simulink model "Motor_ctrl_INST"  (R2024a)
settings: Solver=ode15s  StartTime=0.0  StopTime=1  FixedStep=Ts/10  MaxStep=Tstep  RelTol=1e-3  AbsTol=1e-3  EnableMultiTasking=on
InitFcn:
  | if ~exist('flagwp')
  |     tic
  |     init_sim
  | end
  | mex Motor_ctrl.c User_functions\Src\*.c
StopFcn:
  | if ~exist('flagwp')
  |   elapsed_time=toc
  | end
values from neighbouring files (symbols this model uses):
  accel = 10000    [init_sim.m]
  Bm = 0    [init_sim.m]
  Clarke_inv = [1 0;-0.5 sqrt(3)/2;-0.5 -sqrt(3)/2]    [init_sim.m]
  Ctrl_strategy = 1    [init_sim.m]
  Ctrl_type = 3    [init_sim.m]
  dem = 1    [init_sim.m]
  dT = motorModel.SyreDrive.Converter.dT * 1e-6    [init_sim.m]
  expC = motorModel.IronPMLossMap_dq.expC    [init_sim.m]
  expH = motorModel.IronPMLossMap_dq.expH    [init_sim.m]
  expPM = motorModel.IronPMLossMap_dq.expPM    [init_sim.m]
  fD_pu_norm = motorModel.FluxMapInv_dq.fD_pu_norm    [init_sim.m]
  fD_vct_max = motorModel.FluxMapInv_dq.fD_vct_max    [init_sim.m]
  fD_vct_ref = motorModel.FluxMapInv_dq.fD_vct_ref    [init_sim.m]
  Fm = interp2(Idd,Iqq,Fdd,0,0)    [init_sim.m]
  fQ_pu_norm = motorModel.FluxMapInv_dq.fQ_pu_norm    [init_sim.m]
  fQ_vct_max = motorModel.FluxMapInv_dq.fQ_vct_max    [init_sim.m]
  fQ_vct_ref = motorModel.FluxMapInv_dq.fQ_vct_ref    [init_sim.m]
  HS_ctrl = 1    [init_sim.m]
  Id_dqt = interpn(motorModel.FluxMapInv_dqt.dataF.Fd,motorModel.FluxMapInv_dqt.dataF.Fq,motorModel.FluxMapInv_dqt.dataF.th,motorModel.FluxMapInv_dqt.dataF.Id,Fd_dqt,Fq_dqt,th_dqt,'cubic')    [init_sim.m]
  Id_fe = motorModel.IronPMLossMap_dq.Id    [init_sim.m]
  iD_pu_norm = motorModel.FluxMapInv_dq.iD_pu_norm    [init_sim.m]
  idRef = interp1(abs(MTPA.id+1i*MTPA.iq),MTPA.id,i0)    [init_sim.m]
  InitIntg_d = Fm*cos(th0)    [init_sim.m]
  InitIntg_q = Fm*sin(th0)    [init_sim.m]
  inj_waveform = 1    [init_sim.m]
  Iq_dqt = interpn(motorModel.FluxMapInv_dqt.dataF.Fd,motorModel.FluxMapInv_dqt.dataF.Fq,motorModel.FluxMapInv_dqt.dataF.th,motorModel.FluxMapInv_dqt.dataF.Iq,Fd_dqt,Fq_dqt,th_dqt,'cubic')    [init_sim.m]
  Iq_fe = motorModel.IronPMLossMap_dq.Iq    [init_sim.m]
  iQ_pu_norm = motorModel.FluxMapInv_dq.iQ_pu_norm    [init_sim.m]
  iqRef = interp1(abs(MTPA.id+1i*MTPA.iq),MTPA.iq,i0)    [init_sim.m]
  IronLoss = 1    [init_sim.m]
  J = motorModel.data.J    [init_sim.m]
  motorModelType = motorModel.SyreDrive.modelSetup.motorModelType    [init_sim.m]
  n0 = motorModel.IronPMLossMap_dq.n0    [init_sim.m]
  nRef = 1000    [init_sim.m]
  p = motorModel.data.p    [init_sim.m]
  Pfe_c = motorModel.IronPMLossMap_dq.Pfes_c + motorModel.IronPMLossMap_dq.Pfer_c    [init_sim.m]
  Pfe_h = motorModel.IronPMLossMap_dq.Pfes_h + motorModel.IronPMLossMap_dq.Pfer_h    [init_sim.m]
  Ppm = motorModel.IronPMLossMap_dq.Ppm    [init_sim.m]
  Quad_Maps = 2    [init_sim.m]
  Rs = motorModel.data.Rs    [init_sim.m]
  SS_on = 1    [init_sim.m]
  T_dqt = interpn(motorModel.FluxMapInv_dqt.dataF.Fd,motorModel.FluxMapInv_dqt.dataF.Fq,motorModel.FluxMapInv_dqt.dataF.th,motorModel.FluxMapInv_dqt.dataF.T,Fd_dqt,Fq_dqt,th_dqt,'cubic')    [init_sim.m]
  Tf = 0    [init_sim.m]
  th0 = 0    [init_sim.m]
  th_max = max(motorModel.FluxMapInv_dqt.dataF.th,[],'all')    [init_sim.m]
  th_min = min(motorModel.FluxMapInv_dqt.dataF.th,[],'all')    [init_sim.m]
  Ts = 1/motorModel.SyreDrive.Converter.fPWM    [init_sim.m]
  Tv = 0    [init_sim.m]
  VDC = motorModel.data.Vdc    [init_sim.m]
undefined symbols (not defined in the file or in its folder): ACloss, eMotor, interpn, magnitude, sigbuilder_block, T0
libraries: nesl_utility x52, fl_lib x50, ee_lib x14, simulink x7
(part 4 of 4)

== system Motor_ctrl_INST/Motor model/CCG model/Motor Model/Inverse Flux Maps/3D LUTs/Variant Subsystem/PM-SyR ==
  Fdq : Inport
  theta_elt : Inport  Port=2
  Abs3 : Abs  SaturateOnIntegerOverflow=off
  Demux1 : Demux  Outputs=2
  Interpolation Using Prelookup : Interpolation_n-D  NumberOfTableDimensions=3  Table=T_dqt  LookupTableObject=T_th  RequireIndexFractionAsBus=on  InternalRulePriority=Speed
      settings: InputPortMap=u0,u1,u2
  Interpolation Using Prelookup3 : Interpolation_n-D  NumberOfTableDimensions=3  Table=Id_dqt  RequireIndexFractionAsBus=on  InternalRulePriority=Speed
      settings: InputPortMap=u0,u1,u2
  Interpolation Using Prelookup4 : Interpolation_n-D  NumberOfTableDimensions=3  Table=Iq_dqt  RequireIndexFractionAsBus=on  InternalRulePriority=Speed
      settings: InputPortMap=u0,u1,u2
  MATLAB Function2 : MATLAB Function  TreatAsAtomicUnit=on
  Mux1 : Mux  Inputs=2
  Prelookup1 : PreLookup  BreakpointsData=Fd_v  OutputSelection=Index and fraction as bus  ExtrapMethod=Linear
  Prelookup2 : PreLookup  BreakpointsData=Fq_v  OutputSelection=Index and fraction as bus  ExtrapMethod=Linear
  Prelookup6 : PreLookup  BreakpointsData=th_v  OutputSelection=Index and fraction as bus  ExtrapMethod=Linear
  Product : Product
  Product6 : Product
  Sign2 : Signum
  th_lim : Saturate  UpperLimit=th_max  LowerLimit=th_min  ZeroCross=off
  idq : Outport
  T : Outport  Port=2
  wires:
  Sign2/1 -> Product6/1, Product/1
  Interpolation Using Prelookup3/1 -> Product/2
  ? -> ?
  theta_elt/1 -> MATLAB Function2/1(th_rad)
  Product/1 -> Mux1/1
  Interpolation Using Prelookup4/1 -> Mux1/2
  Product6/1 -> T/1
  Abs3/1 -> Prelookup1/1  "fd"
  MATLAB Function2/1(th_deg) -> th_lim/1
  [bus_d] -> Interpolation Using Prelookup3/2
  [bus_d] -> Interpolation Using Prelookup4/2
  Prelookup1/1 -> [bus_d]
  [bus_q] -> Interpolation Using Prelookup/1
  Demux1/2 -> Prelookup2/1  "fq"
  [bus_th] -> Interpolation Using Prelookup/3
  [bus_q] -> Interpolation Using Prelookup4/1
  [bus_d] -> Interpolation Using Prelookup/2
  [bus_q] -> Interpolation Using Prelookup3/1
  [bus_th] -> Interpolation Using Prelookup4/3
  Demux1/1 -> Sign2/1, Abs3/1  "fd"
  th_lim/1 -> Prelookup6/1
  Prelookup6/1 -> [bus_th]
  [bus_th] -> Interpolation Using Prelookup3/3
  Prelookup2/1 -> [bus_q]
  Mux1/1 -> idq/1
  Fdq/1 -> Demux1/1
  Interpolation Using Prelookup/1 -> Product6/2

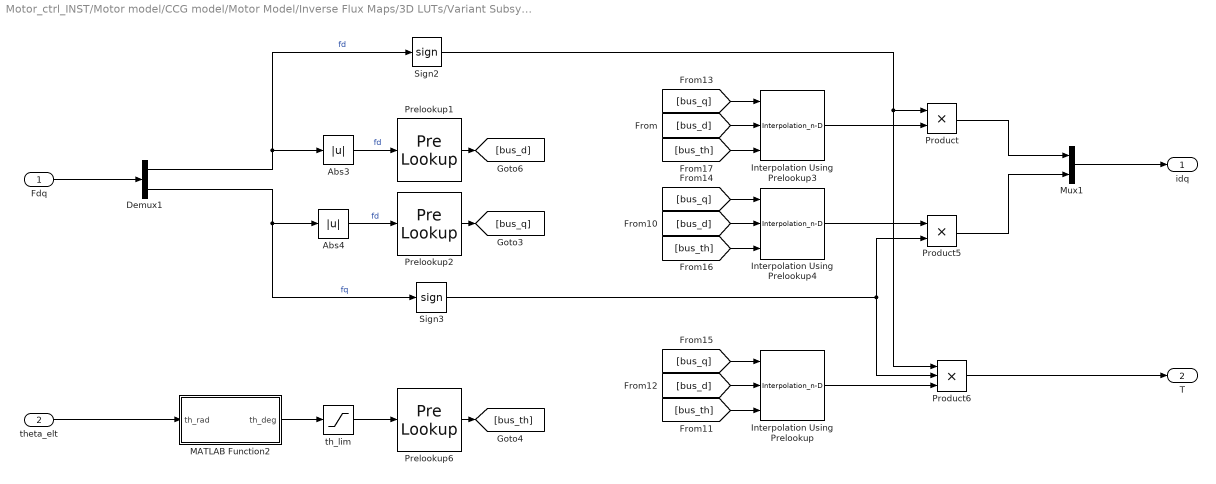
== system Motor_ctrl_INST/Motor model/CCG model/Motor Model/Inverse Flux Maps/3D LUTs/Variant Subsystem/SyR ==
  Fdq : Inport
  theta_elt : Inport  Port=2
  Abs3 : Abs  SaturateOnIntegerOverflow=off
  Abs4 : Abs  SaturateOnIntegerOverflow=off
  Demux1 : Demux  Outputs=2
  Interpolation Using Prelookup : Interpolation_n-D  NumberOfTableDimensions=3  Table=T_dqt  LookupTableObject=T_th  RequireIndexFractionAsBus=on  InternalRulePriority=Speed
      settings: InputPortMap=u0,u1,u2
  Interpolation Using Prelookup3 : Interpolation_n-D  NumberOfTableDimensions=3  Table=Id_dqt  RequireIndexFractionAsBus=on  InternalRulePriority=Speed
      settings: InputPortMap=u0,u1,u2
  Interpolation Using Prelookup4 : Interpolation_n-D  NumberOfTableDimensions=3  Table=Iq_dqt  RequireIndexFractionAsBus=on  InternalRulePriority=Speed
      settings: InputPortMap=u0,u1,u2
  MATLAB Function2 : MATLAB Function  TreatAsAtomicUnit=on
  Mux1 : Mux  Inputs=2
  Prelookup1 : PreLookup  BreakpointsData=Fd_v  OutputSelection=Index and fraction as bus  ExtrapMethod=Linear
  Prelookup2 : PreLookup  BreakpointsData=Fq_v  OutputSelection=Index and fraction as bus  ExtrapMethod=Linear
  Prelookup6 : PreLookup  BreakpointsData=th_v  OutputSelection=Index and fraction as bus  ExtrapMethod=Linear
  Product : Product
  Product5 : Product
  Product6 : Product  Inputs=3
  Sign2 : Signum
  Sign3 : Signum
  th_lim : Saturate  UpperLimit=th_max  LowerLimit=th_min  ZeroCross=off
  idq : Outport
  T : Outport  Port=2
  wires:
  th_lim/1 -> Prelookup6/1
  [bus_q] -> Interpolation Using Prelookup3/1
  Demux1/1 -> Sign2/1, Abs3/1  "fd"
  Prelookup6/1 -> [bus_th]
  Prelookup2/1 -> [bus_q]
  [bus_th] -> Interpolation Using Prelookup4/3
  [bus_q] -> Interpolation Using Prelookup4/1
  Fdq/1 -> Demux1/1
  [bus_q] -> Interpolation Using Prelookup/1
  [bus_th] -> Interpolation Using Prelookup/3
  [bus_d] -> Interpolation Using Prelookup4/2
  [bus_d] -> Interpolation Using Prelookup/2
  Demux1/2 -> Sign3/1, Abs4/1  "fq"
  Prelookup1/1 -> [bus_d]
  theta_elt/1 -> MATLAB Function2/1(th_rad)
  [bus_th] -> Interpolation Using Prelookup3/3
  [bus_d] -> Interpolation Using Prelookup3/2
  MATLAB Function2/1(th_deg) -> th_lim/1
  Abs3/1 -> Prelookup1/1  "fd"
  Abs4/1 -> Prelookup2/1  "fd"
  Interpolation Using Prelookup3/1 -> Product/2
  Sign2/1 -> Product6/1, Product/1
  Interpolation Using Prelookup4/1 -> Product5/1
  Sign3/1 -> Product6/2, Product5/2
  Product/1 -> Mux1/1
  Product5/1 -> Mux1/2
  Mux1/1 -> idq/1
  Interpolation Using Prelookup/1 -> Product6/3
  Product6/1 -> T/1

== system Motor_ctrl_INST/Motor model/CCG model/Motor Model/Iron Losses Maps/Iron Losses/Iron loss Maps/Speed Adaptation ==
  n_m : Inport
  Constant : Constant  Value=n0
  Constant1 : Constant  Value=expC
  Constant2 : Constant  Value=expH
  Constant3 : Constant  Value=expPM
  Divide : Product  Inputs=*/
  Math Function : Math  Operator=pow  SignedPower=on
  Math Function1 : Math  Operator=pow  SignedPower=on
  Math Function2 : Math  Operator=pow  SignedPower=on
  H : Outport
  C : Outport  Port=2
  PM : Outport  Port=3
  wires:
  Math Function2/1 -> PM/1
  Math Function/1 -> H/1
  Constant1/1 -> Math Function1/2
  Divide/1 -> Math Function/1, Math Function1/1, Math Function2/1
  Math Function1/1 -> C/1
  Constant/1 -> Divide/2
  Constant2/1 -> Math Function/2
  Constant3/1 -> Math Function2/2
  n_m/1 -> Divide/1

== system Motor_ctrl_INST/Motor model/CCG model/Motor Model/Inverse Flux Maps/2D LUT/dq Model/IPM/Torque calculation ==
  Idq : Inport
  Fdq : Inport  Port=2
  Add : Sum  Inputs=+-
  Demux1 : Demux  Outputs=2
  Demux3 : Demux  Outputs=2
  Gain2 : Gain  Gain=1.5*p
  Product : Product
  Product1 : Product
  Tm : Outport
  wires:
  Demux1/1 -> Product/1
  Product/1 -> Add/1
  Demux3/1 -> Product1/2
  Demux3/2 -> Product/2
  Demux1/2 -> Product1/1
  Product1/1 -> Add/2
  Fdq/1 -> Demux1/1
  Add/1 -> Gain2/1
  Idq/1 -> Demux3/1
  Gain2/1 -> Tm/1

== system Motor_ctrl_INST/Motor model/CCG model/Motor Model/Inverse Flux Maps/2D LUT/dq Model/PM-SyR/Torque calculation ==
  Idq : Inport
  Fdq : Inport  Port=2
  Add : Sum  Inputs=+-
  Demux1 : Demux  Outputs=2
  Demux3 : Demux  Outputs=2
  Gain2 : Gain  Gain=1.5*p
  Product : Product
  Product1 : Product
  Tm : Outport
  wires:
  Demux1/1 -> Product/1
  Product/1 -> Add/1
  Demux3/1 -> Product1/2
  Demux3/2 -> Product/2
  Demux1/2 -> Product1/1
  Product1/1 -> Add/2
  Fdq/1 -> Demux1/1
  Add/1 -> Gain2/1
  Idq/1 -> Demux3/1
  Gain2/1 -> Tm/1

== system Motor_ctrl_INST/Motor model/CCG model/Motor Model/Inverse Flux Maps/2D LUT/dq Model/SyR/Torque calculation ==
  Idq : Inport
  Fdq : Inport  Port=2
  Add : Sum  Inputs=+-
  Demux1 : Demux  Outputs=2
  Demux3 : Demux  Outputs=2
  Gain2 : Gain  Gain=1.5*p
  Product : Product
  Product1 : Product
  Tm : Outport
  wires:
  Demux1/1 -> Product/1
  Product/1 -> Add/1
  Demux3/1 -> Product1/2
  Demux3/2 -> Product/2
  Demux1/2 -> Product1/1
  Product1/1 -> Add/2
  Fdq/1 -> Demux1/1
  Add/1 -> Gain2/1
  Idq/1 -> Demux3/1
  Gain2/1 -> Tm/1

== matlab function Motor_ctrl_INST/Motor Model/Motor Model/Inverse Flux Maps/3D LUTs/Variant Subsystem/PM-SyR/MATLAB Function2 ==
  data: th_rad input; th_deg output
function th_deg = fcn(th_rad)

th_deg=th_rad*180/pi;

while th_deg>360
    th_deg=th_deg-360;
end

while th_deg<0
    th_deg=th_deg+360;
end

== matlab function Motor_ctrl_INST/Motor model/CCG model/Motor Model/Inverse Flux Maps/3D LUTs/Variant Subsystem/IPM/MATLAB Function2 ==
  data: th_rad input; th_deg output
function th_deg = fcn(th_rad)

th_deg=th_rad*180/pi;

while th_deg>360
    th_deg=th_deg-360;
end

while th_deg<0
    th_deg=th_deg+360;
end

== matlab function Motor_ctrl_INST/Motor Model/Motor Model/Inverse Flux Maps/3D LUTs/Variant Subsystem/IPM/MATLAB Function2 ==
  data: th_rad input; th_deg output
function th_deg = fcn(th_rad)

th_deg=th_rad*180/pi;

while th_deg>360
    th_deg=th_deg-360;
end

while th_deg<0
    th_deg=th_deg+360;
end

== matlab function Motor_ctrl_INST/Motor Model/Motor Model/Iron Losses Maps/Iron Losses/Iron loss Maps/Stator Voltage Eqaution1 ==
  data: idq_m input; Quad_Maps input; idq_out output
function idq_out = fcn(idq_m, Quad_Maps)

idq_out = [0; 0];

switch(Quad_Maps)
    case 0 %SyR
        idq_out(1) = abs(idq_m(1));
        idq_out(2) = abs(idq_m(2));
    case 1  %PM-SyR
        idq_out(1) = abs(idq_m(1));
        idq_out(2) = idq_m(2);
    case 2  %PM  
        idq_out(1) = idq_m(1);
        idq_out(2) = abs(idq_m(2));
end

end

== matlab function Motor_ctrl_INST/Motor Model/Motor Model/Iron Losses Maps/Iron Losses/Iron loss Maps/MATLAB Function1 ==
  data: P input; Id_fe output; Fdq input; n input; p input; Iq_fe output
function [Id_fe,Iq_fe] = fcn(P,Fdq,n,p)

Id_fe = 0;
Iq_fe = 0; 

if(n>0)
    tmp1 = (n*pi*p)/30;
    tmp2 = Fdq(1)*Fdq(1)+Fdq(2)*Fdq(2);
    tmp3 = tmp1*tmp2;
    Id_fe = (P/tmp3)*(-Fdq(2));
    Iq_fe = (P/tmp3)*(Fdq(1));

   
end    

end

== matlab function Motor_ctrl_INST/Motor model/CCG model/Motor Model/Inverse Flux Maps/3D LUTs/Variant Subsystem/PM-SyR/MATLAB Function2 ==
  data: th_rad input; th_deg output
function th_deg = fcn(th_rad)

th_deg=th_rad*180/pi;

while th_deg>360
    th_deg=th_deg-360;
end

while th_deg<0
    th_deg=th_deg+360;
end

== matlab function Motor_ctrl_INST/Motor Model/Motor Model/Inverse Flux Maps/3D LUTs/Variant Subsystem/SyR/MATLAB Function2 ==
  data: th_rad input; th_deg output
function th_deg = fcn(th_rad)

th_deg=th_rad*180/pi;

while th_deg>360
    th_deg=th_deg-360;
end

while th_deg<0
    th_deg=th_deg+360;
end

== matlab function Motor_ctrl_INST/Motor model/CCG model/Motor Model/Inverse Flux Maps/3D LUTs/Variant Subsystem/SyR/MATLAB Function2 ==
  data: th_rad input; th_deg output
function th_deg = fcn(th_rad)

th_deg=th_rad*180/pi;

while th_deg>360
    th_deg=th_deg-360;
end

while th_deg<0
    th_deg=th_deg+360;
end

== matlab function Motor_ctrl_INST/Motor model/CCG model/Motor Model/Iron Losses Maps/Iron Losses/Iron loss Maps/MATLAB Function1 ==
  data: P input; Id_fe output; Fdq input; n input; p input; Iq_fe output
function [Id_fe,Iq_fe] = fcn(P,Fdq,n,p)

Id_fe = 0;
Iq_fe = 0; 

if(n>0)
    tmp1 = (n*pi*p)/30;
    tmp2 = Fdq(1)*Fdq(1)+Fdq(2)*Fdq(2);
    tmp3 = tmp1*tmp2;
    Id_fe = (P/tmp3)*(-Fdq(2));
    Iq_fe = (P/tmp3)*(Fdq(1));

   
end    

end

== matlab function Motor_ctrl_INST/Motor model/CCG model/Motor Model/Iron Losses Maps/Iron Losses/Iron loss Maps/Stator Voltage Eqaution1 ==
  data: idq_m input; Quad_Maps input; idq_out output
function idq_out = fcn(idq_m, Quad_Maps)

idq_out = [0; 0];

switch(Quad_Maps)
    case 0 %SyR
        idq_out(1) = abs(idq_m(1));
        idq_out(2) = abs(idq_m(2));
    case 1  %PM-SyR
        idq_out(1) = abs(idq_m(1));
        idq_out(2) = idq_m(2);
    case 2  %PM  
        idq_out(1) = idq_m(1);
        idq_out(2) = abs(idq_m(2));
end

end
